simulink library "ammclib_bam_S32K14x"  (R2016a)
settings: Solver=VariableStepAuto  SolverMode=SingleTasking  StartTime=0.0  StopTime=10.0  RelTol=1e-3
undefined symbols (not defined in the file or in its folder): f16A1, f16A2, f16ADCMaxError, f16B0, f16B1, f16B2, f16C1, f16CC1, f16CC1sc, f16CC1sc_D, f16CC1sc_Q, f16CC2, f16CC2sc, f16CC2sc_D, f16CC2sc_Q, f16DerivGain, f16EGain, f16FiltCoef, f16HystOff, f16HystOn, f16IGain, f16IntegGain, f16IntegGainFW, f16IntegGainQ, f16Kd, f16Kq, f16Limit, f16LowerLimit, f16LowerLimit_D, f16LowerLimit_Q, f16LowerLimitFW, f16LowerLimitQ, f16ModIndex, f16OutValOff, f16OutValOn, f16PropGain, f16PropGainFW, f16PropGainQ, f16RampDown, f16RampUp, f16UGain, f16UpperLimit, f16UpperLimit_D, f16UpperLimit_Q, f16UpperLimitFW, f16UpperLimitQ, f16WIGain, f32A1, f32A2, f32ADCMaxError, f32B0, f32B1, f32B2, f32C1, f32CC1, f32CC1sc, f32CC1sc_D, f32CC1sc_Q, f32CC2, f32CC2sc ... (+114)
(part 15 of 22)

== system ammclib_bam_S32K14x/GMCLIB/FLT ==
  GMCLIB_BetaProjection3Ph_FLT : Subsystem  TreatAsAtomicUnit=on  mask(GMCLIB_BetaProjection3Ph_FLT){}
      mask help: 3-phase Beta-projection transformation in single precision floating-point implementation. Refer to the AMMCLIB User's Guide for further details.
      mask init: same as ammclib_bam_S32K14x/GDFLIB/F16/GDFLIB_FilterFIR_F16
      settings: RTWSystemCode=Inline
      mask Help: web([fileparts(which('ammclib_bam_S32K14x.slx')) '/../doc/S32K14XMCLUG.pdf'], '-browser')
      mask Display: pos = get_param(gcb, 'Position');width = pos(3) - pos(1); height = pos(4) - pos(2);tX=width/2;tY=height - 8;color('black');text(tX,tY, 'GMCLIB_BetaProjection3Ph_FLT', 'horizontalAlignment', 'center');
  GMCLIB_BetaProjection_FLT : Subsystem  TreatAsAtomicUnit=on  mask(GMCLIB_BetaProjection_FLT){}
      mask help: Beta Projection transformation 3ph -> 2ph in single precision floating-point implementation. Refer to the AMMCLIB User's Guide for further details.
      mask init: same as ammclib_bam_S32K14x/GDFLIB/F16/GDFLIB_FilterFIR_F16
      settings: RTWSystemCode=Inline
      mask Help: web([fileparts(which('ammclib_bam_S32K14x.slx')) '/../doc/S32K14XMCLUG.pdf'], '-browser')
      mask Display: pos = get_param(gcb, 'Position');width = pos(3) - pos(1); height = pos(4) - pos(2);tX=width/2;tY=height - 8;color('black');text(tX,tY, 'GMCLIB_BetaProjection_FLT', 'horizontalAlignment', 'center');
  GMCLIB_ClarkInv_FLT : Subsystem  TreatAsAtomicUnit=on  mask(GMCLIB_ClarkInv_FLT){}
      mask help: Inverse Clarke transformation 2ph -> 3ph in single precision floating-point implementation. Refer to the AMMCLIB User's Guide for further details.
      mask init: same as ammclib_bam_S32K14x/GDFLIB/F16/GDFLIB_FilterFIR_F16
      settings: RTWSystemCode=Inline
      mask Help: web([fileparts(which('ammclib_bam_S32K14x.slx')) '/../doc/S32K14XMCLUG.pdf'], '-browser')
      mask Display: pos = get_param(gcb, 'Position');width = pos(3) - pos(1); height = pos(4) - pos(2);tX=width/2;tY=height - 8;color('black');text(tX,tY, 'GMCLIB_ClarkInv_FLT', 'horizontalAlignment', 'center');
  GMCLIB_Clark_FLT : Subsystem  TreatAsAtomicUnit=on  mask(GMCLIB_Clark_FLT){}
      mask help: Clarke transformation 3ph -> 2ph in single precision floating-point implementation. Refer to the AMMCLIB User's Guide for further details.
      mask init: same as ammclib_bam_S32K14x/GDFLIB/F16/GDFLIB_FilterFIR_F16
      settings: RTWSystemCode=Inline
      mask Help: web([fileparts(which('ammclib_bam_S32K14x.slx')) '/../doc/S32K14XMCLUG.pdf'], '-browser')
      mask Display: pos = get_param(gcb, 'Position');width = pos(3) - pos(1); height = pos(4) - pos(2);tX=width/2;tY=height - 8;color('black');text(tX,tY, 'GMCLIB_Clark_FLT', 'horizontalAlignment', 'center');
  GMCLIB_DecouplingPMSM_FLT : Subsystem  TreatAsAtomicUnit=on  mask(GMCLIB_DecouplingPMSM_FLT){showStates=Hide (faster execution), fltLD=0, fltLQ=0}
      mask prompts: showStates "Show internal states"; fltLD "fltLD (D component of motor inductance [H])"; fltLQ "fltLQ (Q component of motor inductance [H])"
      mask help: Decoupling of d and q axis of PMSM model in single precision floating-point implementation. Refer to the AMMCLIB User's Guide for further details.
      mask init:
      | if ~evalin('base','exist(''tS8'',''var'')')
      |   if (2 ~= exist('SWLIBS_Typedefs.mat','file'))
      |       error('File SWLIBS_Typedefs.mat is not on the Matlab path. Please add the AMMCLIB "bam" folder in the Matlab Search Path.');
      |   else
      |       evalin('base', 'load(''SWLIBS_Typedefs.mat'')');
      |   end
      | end
      | if showStates == 1
      |     % hidden state variables
      |     if strcmp(get_param([gcb '/fltLD'], 'BlockType'), 'Inport')
      |         posblk = get_param(gcb, 'Position');
      | 
      |         pos = get_param(    [gcb, '/fltLD'], 'Position');
      |         orient = get_param( [gcb, '/fltLD'], 'Orientation');
      |         delete_block(       [gcb, '/fltLD']);
      |         add_block('built-in/Ground', [gcb, '/fltLD'], 'Position', pos, 'Orientation', orient);
      | 
      |         pos = get_param(    [gcb, '/fltLQ'], 'Position');
      |         orient = get_param( [gcb, '/fltLQ'], 'Orientation');
      |         delete_block(       [gcb, '/fltLQ']);
      |         add_block('built-in/Ground', [gcb, '/fltLQ'], 'Position', pos, 'Orientation', orient);
      | 
      | 
      | 
      |         set_param([gcb '/pUdq'], 'Port', '1');
      |         set_param([gcb '/pIdq'], 'Port', '2');
      |         set_param([gcb '/fltAngularVel'], 'Port', '3');
      | 
      |         set_param([gcb '/pUdqDec'], 'Port', '1');
      | 
      |         set_param(gcb,'MaskEnables',{'on','on','on'});
      | 
      |         if (posblk(4) - posblk(2)) > 100
      |           height = 100;
      |           set_param(gcb,'Position',[posblk(1), posblk(2), posblk(3), posblk(2)+height])
      |         end
      |     end
      | else
      |     % shown state variables
      |     if strcmp(get_param([gcb '/fltLD'], 'BlockType'), 'Ground')
      |         posblk = get_param(gcb, 'Position');
      | 
      |         pos = get_param(    [gcb, '/fltLD'], 'Position');
      |         orient = get_param( [gcb, '/fltLD'], 'Orientation');
      |         delete_block(       [gcb, '/fltLD']);
      |         add_block('built-in/Inport', [gcb, '/fltLD'], 'Position', pos, 'Orientation', orient, 'OutDataTypeStr', 'single');
      | 
      |         pos = get_param(    [gcb, '/fltLQ'], 'Position');
      |         orient = get_param( [gcb, '/fltLQ'], 'Orientation');
      |         delete_block(       [gcb, '/fltLQ']);
      |         add_block('built-in/Inport', [gcb, '/fltLQ'], 'Position', pos, 'Orientation', orient, 'OutDataTypeStr', 'single');
      | 
      | 
      | 
      |         set_param([gcb '/pUdq'], 'Port', '1');
      |         set_param([gcb '/pIdq'], 'Port', '2');
      |         set_param([gcb '/fltAngularVel'], 'Port', '3');
      |         set_param([gcb '/fltLD'], 'Port', '4');
      |         set_param([gcb '/fltLQ'], 'Port', '5');
      | 
      |         set_param([gcb '/pUdqDec'], 'Port', '1');
      | 
      |         set_param(gcb,'MaskEnables',{'on','off','off'});
      | 
      |         if (posblk(4) - posblk(2)) < 150
      |           height = 150;
      |           set_param(gcb,'Position',[posblk(1), posblk(2), posblk(3), posblk(2)+height])
      |         end
      |     end
      | end
      settings: RTWSystemCode=Inline
      mask Help: web([fileparts(which('ammclib_bam_S32K14x.slx')) '/../doc/S32K14XMCLUG.pdf'], '-browser')
      mask TypeOptions showStates: Hide (faster execution) | Show (allows debugging; connect feedback loops manually)
      mask Callback showStates:
      | maskStr = get_param(gcb,'showStates');
      | if strcmp(maskStr,'Hide (faster execution)'),
      |     set_param(gcb,'MaskEnables',{'on','on','on'});
      | else
      |     set_param(gcb,'MaskEnables',{'on','off','off'});
      | end
      mask Display:
      | color('black');
      | pos = get_param(gcb, 'Position');
      | width = pos(3) - pos(1);
      | height = pos(4) - pos(2);
      | tX=width/2;
      | tY=height - 8;
      | color('black');
      | text(tX,tY, 'GMCLIB_DecouplingPMSM_FLT', 'horizontalAlignment', 'center');
      | if showStates == 2
      |   color('red');
      |   text(tX,tY - 20, ['debugging mode' char(13) char(10) '(limited performance)'], 'horizontalAlignment', 'center');
      | end
  GMCLIB_ElimDcBusRip_FLT : Subsystem  TreatAsAtomicUnit=on  mask(GMCLIB_ElimDcBusRip_FLT){showStates=Hide (faster execution), fltModIndex=0}
      mask prompts: showStates "Show internal states"; fltModIndex "fltModIndex (Inverse Modulation Index)"
      mask help: DC Bus voltage ripple elimination function in single precision floating-point implementation. Refer to the AMMCLIB User's Guide for further details.
      mask init:
      | if ~evalin('base','exist(''tS8'',''var'')')
      |   if (2 ~= exist('SWLIBS_Typedefs.mat','file'))
      |       error('File SWLIBS_Typedefs.mat is not on the Matlab path. Please add the AMMCLIB "bam" folder in the Matlab Search Path.');
      |   else
      |       evalin('base', 'load(''SWLIBS_Typedefs.mat'')');
      |   end
      | end
      | if showStates == 1
      |     % hidden state variables
      |     if strcmp(get_param([gcb '/fltModIndex'], 'BlockType'), 'Inport')
      |         posblk = get_param(gcb, 'Position');
      | 
      |         pos = get_param(    [gcb, '/fltModIndex'], 'Position');
      |         orient = get_param( [gcb, '/fltModIndex'], 'Orientation');
      |         delete_block(       [gcb, '/fltModIndex']);
      |         add_block('built-in/Ground', [gcb, '/fltModIndex'], 'Position', pos, 'Orientation', orient);
      | 
      | 
      | 
      |         set_param([gcb '/pIn'], 'Port', '1');
      |         set_param([gcb '/fltArgDcBusMsr'], 'Port', '2');
      | 
      |         set_param([gcb '/pOut'], 'Port', '1');
      | 
      |         set_param(gcb,'MaskEnables',{'on','on'});
      | 
      |         if (posblk(4) - posblk(2)) > 75
      |           height = 75;
      |           set_param(gcb,'Position',[posblk(1), posblk(2), posblk(3), posblk(2)+height])
      |         end
      |     end
      | else
      |     % shown state variables
      |     if strcmp(get_param([gcb '/fltModIndex'], 'BlockType'), 'Ground')
      |         posblk = get_param(gcb, 'Position');
      | 
      |         pos = get_param(    [gcb, '/fltModIndex'], 'Position');
      |         orient = get_param( [gcb, '/fltModIndex'], 'Orientation');
      |         delete_block(       [gcb, '/fltModIndex']);
      |         add_block('built-in/Inport', [gcb, '/fltModIndex'], 'Position', pos, 'Orientation', orient, 'OutDataTypeStr', 'single');
      | 
      | 
      | 
      |         set_param([gcb '/pIn'], 'Port', '1');
      |         set_param([gcb '/fltArgDcBusMsr'], 'Port', '2');
      |         set_param([gcb '/fltModIndex'], 'Port', '3');
      | 
      |         set_param([gcb '/pOut'], 'Port', '1');
      | 
      |         set_param(gcb,'MaskEnables',{'on','off'});
      | 
      |         if (posblk(4) - posblk(2)) < 100
      |           height = 100;
      |           set_param(gcb,'Position',[posblk(1), posblk(2), posblk(3), posblk(2)+height])
      |         end
      |     end
      | end
      settings: RTWSystemCode=Inline
      mask Help: web([fileparts(which('ammclib_bam_S32K14x.slx')) '/../doc/S32K14XMCLUG.pdf'], '-browser')
      mask TypeOptions showStates: Hide (faster execution) | Show (allows debugging; connect feedback loops manually)
      mask Callback showStates:
      | maskStr = get_param(gcb,'showStates');
      | if strcmp(maskStr,'Hide (faster execution)'),
      |     set_param(gcb,'MaskEnables',{'on','on'});
      | else
      |     set_param(gcb,'MaskEnables',{'on','off'});
      | end
      mask Display:
      | color('black');
      | pos = get_param(gcb, 'Position');
      | width = pos(3) - pos(1);
      | height = pos(4) - pos(2);
      | tX=width/2;
      | tY=height - 8;
      | color('black');
      | text(tX,tY, 'GMCLIB_ElimDcBusRip_FLT', 'horizontalAlignment', 'center');
      | if showStates == 2
      |   color('red');
      |   text(tX,tY - 20, ['debugging mode' char(13) char(10) '(limited performance)'], 'horizontalAlignment', 'center');
      | end
  GMCLIB_ParkInv_FLT : Subsystem  TreatAsAtomicUnit=on  mask(GMCLIB_ParkInv_FLT){}
      mask help: Inverse Park transformation 2ph rotational -> 2ph stationary in single precision floating-point implementation. Refer to the AMMCLIB User's Guide for further details.
      mask init: same as ammclib_bam_S32K14x/GDFLIB/F16/GDFLIB_FilterFIR_F16
      settings: RTWSystemCode=Inline
      mask Help: web([fileparts(which('ammclib_bam_S32K14x.slx')) '/../doc/S32K14XMCLUG.pdf'], '-browser')
      mask Display: pos = get_param(gcb, 'Position');width = pos(3) - pos(1); height = pos(4) - pos(2);tX=width/2;tY=height - 8;color('black');text(tX,tY, 'GMCLIB_ParkInv_FLT', 'horizontalAlignment', 'center');
  GMCLIB_Park_FLT : Subsystem  TreatAsAtomicUnit=on  mask(GMCLIB_Park_FLT){}
      mask help: Park transformation 2ph stationary -> 2ph rotational in single precision floating-point implementation. Refer to the AMMCLIB User's Guide for further details.
      mask init: same as ammclib_bam_S32K14x/GDFLIB/F16/GDFLIB_FilterFIR_F16
      settings: RTWSystemCode=Inline
      mask Help: web([fileparts(which('ammclib_bam_S32K14x.slx')) '/../doc/S32K14XMCLUG.pdf'], '-browser')
      mask Display: pos = get_param(gcb, 'Position');width = pos(3) - pos(1); height = pos(4) - pos(2);tX=width/2;tY=height - 8;color('black');text(tX,tY, 'GMCLIB_Park_FLT', 'horizontalAlignment', 'center');
  GMCLIB_PwmIct_FLT : Subsystem  TreatAsAtomicUnit=on  mask(GMCLIB_PwmIct_FLT){}
      mask help: General Sinusoidal PWM in single precision floating-point implementation. Refer to the AMMCLIB User's Guide for further details.
      mask init: same as ammclib_bam_S32K14x/GDFLIB/F16/GDFLIB_FilterFIR_F16
      settings: RTWSystemCode=Inline
      mask Help: web([fileparts(which('ammclib_bam_S32K14x.slx')) '/../doc/S32K14XMCLUG.pdf'], '-browser')
      mask Display: pos = get_param(gcb, 'Position');width = pos(3) - pos(1); height = pos(4) - pos(2);tX=width/2;tY=height - 8;color('black');text(tX,tY, 'GMCLIB_PwmIct_FLT', 'horizontalAlignment', 'center');
  GMCLIB_SvmSci_FLT : Subsystem  TreatAsAtomicUnit=on  mask(GMCLIB_SvmSci_FLT){}
      mask help: General Sinusoidal Modulation with Injection of Third Harmonic in single precision floating-point implementation. Refer to the AMMCLIB User's Guide for further details.
      mask init: same as ammclib_bam_S32K14x/GDFLIB/F16/GDFLIB_FilterFIR_F16
      settings: RTWSystemCode=Inline
      mask Help: web([fileparts(which('ammclib_bam_S32K14x.slx')) '/../doc/S32K14XMCLUG.pdf'], '-browser')
      mask Display: pos = get_param(gcb, 'Position');width = pos(3) - pos(1); height = pos(4) - pos(2);tX=width/2;tY=height - 8;color('black');text(tX,tY, 'GMCLIB_SvmSci_FLT', 'horizontalAlignment', 'center');
  GMCLIB_SvmStd_FLT : Subsystem  TreatAsAtomicUnit=on  mask(GMCLIB_SvmStd_FLT){}
      mask help: Standard Space Vector Modulation in single precision floating-point implementation. Refer to the AMMCLIB User's Guide for further details.
      mask init: same as ammclib_bam_S32K14x/GDFLIB/F16/GDFLIB_FilterFIR_F16
      settings: RTWSystemCode=Inline
      mask Help: web([fileparts(which('ammclib_bam_S32K14x.slx')) '/../doc/S32K14XMCLUG.pdf'], '-browser')
      mask Display: pos = get_param(gcb, 'Position');width = pos(3) - pos(1); height = pos(4) - pos(2);tX=width/2;tY=height - 8;color('black');text(tX,tY, 'GMCLIB_SvmStd_FLT', 'horizontalAlignment', 'center');
  GMCLIB_SvmU0n_FLT : Subsystem  TreatAsAtomicUnit=on  mask(GMCLIB_SvmU0n_FLT){}
      mask help: Special Space Vector Modulation with O_000 Nulls in single precision floating-point implementation. Refer to the AMMCLIB User's Guide for further details.
      mask init: same as ammclib_bam_S32K14x/GDFLIB/F16/GDFLIB_FilterFIR_F16
      settings: RTWSystemCode=Inline
      mask Help: web([fileparts(which('ammclib_bam_S32K14x.slx')) '/../doc/S32K14XMCLUG.pdf'], '-browser')
      mask Display: pos = get_param(gcb, 'Position');width = pos(3) - pos(1); height = pos(4) - pos(2);tX=width/2;tY=height - 8;color('black');text(tX,tY, 'GMCLIB_SvmU0n_FLT', 'horizontalAlignment', 'center');
  GMCLIB_SvmU7n_FLT : Subsystem  TreatAsAtomicUnit=on  mask(GMCLIB_SvmU7n_FLT){}
      mask help: Special Space Vector Modulation with O_111 Ones in single precision floating-point implementation. Refer to the AMMCLIB User's Guide for further details.
      mask init: same as ammclib_bam_S32K14x/GDFLIB/F16/GDFLIB_FilterFIR_F16
      settings: RTWSystemCode=Inline
      mask Help: web([fileparts(which('ammclib_bam_S32K14x.slx')) '/../doc/S32K14XMCLUG.pdf'], '-browser')
      mask Display: pos = get_param(gcb, 'Position');width = pos(3) - pos(1); height = pos(4) - pos(2);tX=width/2;tY=height - 8;color('black');text(tX,tY, 'GMCLIB_SvmU7n_FLT', 'horizontalAlignment', 'center');
  GMCLIB_VRot_FLT : Subsystem  TreatAsAtomicUnit=on  mask(GMCLIB_VRot_FLT){}
      mask help: Vector rotation in single precision floating-point implementation.
      mask init: same as ammclib_bam_S32K14x/GDFLIB/F16/GDFLIB_FilterFIR_F16
      settings: RTWSystemCode=Inline
      mask Help: web([fileparts(which('ammclib_bam_S32K14x.slx')) '/../doc/S32K14XMCLUG.pdf'], '-browser')
      mask Display: pos = get_param(gcb, 'Position');width = pos(3) - pos(1); height = pos(4) - pos(2);tX=width/2;tY=height - 8;color('black');text(tX,tY, 'GMCLIB_VRot_FLT', 'horizontalAlignment', 'center');
  GMCLIB_VUnit_FLT : Subsystem  TreatAsAtomicUnit=on  mask(GMCLIB_VUnit_FLT){}
      mask help: Vector normalization in single precision floating-point implementation.
      mask init: same as ammclib_bam_S32K14x/GDFLIB/F16/GDFLIB_FilterFIR_F16
      settings: RTWSystemCode=Inline
      mask Help: web([fileparts(which('ammclib_bam_S32K14x.slx')) '/../doc/S32K14XMCLUG.pdf'], '-browser')
      mask Display: pos = get_param(gcb, 'Position');width = pos(3) - pos(1); height = pos(4) - pos(2);tX=width/2;tY=height - 8;color('black');text(tX,tY, 'GMCLIB_VUnit_FLT', 'horizontalAlignment', 'center');
  GMCLIB_Vpol2xy_FLT : Subsystem  TreatAsAtomicUnit=on  mask(GMCLIB_Vpol2xy_FLT){}
      mask help: Transformation of polar coordinate system to Cartesian in single precision floating-point implementation.
      mask init: same as ammclib_bam_S32K14x/GDFLIB/F16/GDFLIB_FilterFIR_F16
      settings: RTWSystemCode=Inline
      mask Help: web([fileparts(which('ammclib_bam_S32K14x.slx')) '/../doc/S32K14XMCLUG.pdf'], '-browser')
      mask Display: pos = get_param(gcb, 'Position');width = pos(3) - pos(1); height = pos(4) - pos(2);tX=width/2;tY=height - 8;color('black');text(tX,tY, 'GMCLIB_Vpol2xy_FLT', 'horizontalAlignment', 'center');
  GMCLIB_Vxy2pol_FLT : Subsystem  TreatAsAtomicUnit=on  mask(GMCLIB_Vxy2pol_FLT){}
      mask help: Transformation of Cartesian coordinate system to polar in single precision floating-point implementation.
      mask init: same as ammclib_bam_S32K14x/GDFLIB/F16/GDFLIB_FilterFIR_F16
      settings: RTWSystemCode=Inline
      mask Help: web([fileparts(which('ammclib_bam_S32K14x.slx')) '/../doc/S32K14XMCLUG.pdf'], '-browser')
      mask Display: pos = get_param(gcb, 'Position');width = pos(3) - pos(1); height = pos(4) - pos(2);tX=width/2;tY=height - 8;color('black');text(tX,tY, 'GMCLIB_Vxy2pol_FLT', 'horizontalAlignment', 'center');

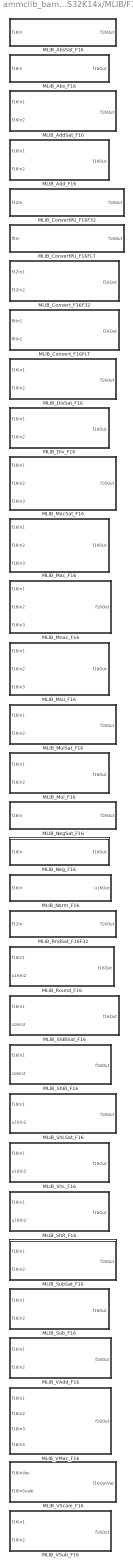
== system ammclib_bam_S32K14x/MLIB/F16 ==
  MLIB_AbsSat_F16 : Subsystem  TreatAsAtomicUnit=on  mask(MLIB_AbsSat_F16){}
      mask help: Saturated absolute value in 16-bit fixed-point fractional implementation. Refer to the AMMCLIB User's Guide for further details.
      mask init: same as ammclib_bam_S32K14x/GDFLIB/F16/GDFLIB_FilterFIR_F16
      settings: RTWSystemCode=Inline
      mask Help: web([fileparts(which('ammclib_bam_S32K14x.slx')) '/../doc/S32K14XMCLUG.pdf'], '-browser')
      mask Display: pos = get_param(gcb, 'Position');width = pos(3) - pos(1); height = pos(4) - pos(2);tX=width/2;tY=height - 8;color('black');text(tX,tY, 'MLIB_AbsSat_F16', 'horizontalAlignment', 'center');
  MLIB_Abs_F16 : Subsystem  TreatAsAtomicUnit=on  mask(MLIB_Abs_F16){}
      mask help: Unsaturated absolute value in 16-bit fixed-point fractional implementation. Refer to the AMMCLIB User's Guide for further details.
      mask init: same as ammclib_bam_S32K14x/GDFLIB/F16/GDFLIB_FilterFIR_F16
      settings: RTWSystemCode=Inline
      mask Help: web([fileparts(which('ammclib_bam_S32K14x.slx')) '/../doc/S32K14XMCLUG.pdf'], '-browser')
      mask Display: pos = get_param(gcb, 'Position');width = pos(3) - pos(1); height = pos(4) - pos(2);tX=width/2;tY=height - 8;color('black');text(tX,tY, 'MLIB_Abs_F16', 'horizontalAlignment', 'center');
  MLIB_AddSat_F16 : Subsystem  TreatAsAtomicUnit=on  mask(MLIB_AddSat_F16){}
      mask help: Saturated addition in 16-bit fixed-point fractional implementation. Refer to the AMMCLIB User's Guide for further details.
      mask init: same as ammclib_bam_S32K14x/GDFLIB/F16/GDFLIB_FilterFIR_F16
      settings: RTWSystemCode=Inline
      mask Help: web([fileparts(which('ammclib_bam_S32K14x.slx')) '/../doc/S32K14XMCLUG.pdf'], '-browser')
      mask Display: pos = get_param(gcb, 'Position');width = pos(3) - pos(1); height = pos(4) - pos(2);tX=width/2;tY=height - 8;color('black');text(tX,tY, 'MLIB_AddSat_F16', 'horizontalAlignment', 'center');
  MLIB_Add_F16 : Subsystem  TreatAsAtomicUnit=on  mask(MLIB_Add_F16){}
      mask help: Unsaturated addition in 16-bit fixed-point fractional implementation.
      mask init: same as ammclib_bam_S32K14x/GDFLIB/F16/GDFLIB_FilterFIR_F16
      settings: RTWSystemCode=Inline
      mask Help: web([fileparts(which('ammclib_bam_S32K14x.slx')) '/../doc/S32K14XMCLUG.pdf'], '-browser')
      mask Display: pos = get_param(gcb, 'Position');width = pos(3) - pos(1); height = pos(4) - pos(2);tX=width/2;tY=height - 8;color('black');text(tX,tY, 'MLIB_Add_F16', 'horizontalAlignment', 'center');
  MLIB_ConvertPU_F16F32 : Subsystem  TreatAsAtomicUnit=on  mask(MLIB_ConvertPU_F16F32){}
      mask help: Conversion of a 32-bit fixed-point fractional value to a 16-bit fixed-point fractional equivalent. Refer to the AMMCLIB User's Guide for further details.
      mask init: same as ammclib_bam_S32K14x/GDFLIB/F16/GDFLIB_FilterFIR_F16
      settings: RTWSystemCode=Inline
      mask Help: web([fileparts(which('ammclib_bam_S32K14x.slx')) '/../doc/S32K14XMCLUG.pdf'], '-browser')
      mask Display: pos = get_param(gcb, 'Position');width = pos(3) - pos(1); height = pos(4) - pos(2);tX=width/2;tY=height - 8;color('black');text(tX,tY, 'MLIB_ConvertPU_F16F32', 'horizontalAlignment', 'center');
  MLIB_ConvertPU_F16FLT : Subsystem  TreatAsAtomicUnit=on  mask(MLIB_ConvertPU_F16FLT){}
      mask help: Conversion of a single precision floating-point value to a 16-bit fixed-point fractional equivalent. Refer to the AMMCLIB User's Guide for further details.
      mask init: same as ammclib_bam_S32K14x/GDFLIB/F16/GDFLIB_FilterFIR_F16
      settings: RTWSystemCode=Inline
      mask Help: web([fileparts(which('ammclib_bam_S32K14x.slx')) '/../doc/S32K14XMCLUG.pdf'], '-browser')
      mask Display: pos = get_param(gcb, 'Position');width = pos(3) - pos(1); height = pos(4) - pos(2);tX=width/2;tY=height - 8;color('black');text(tX,tY, 'MLIB_ConvertPU_F16FLT', 'horizontalAlignment', 'center');
  MLIB_Convert_F16F32 : Subsystem  TreatAsAtomicUnit=on  mask(MLIB_Convert_F16F32){}
      mask help: Scaled conversion of a 32-bit fixed-point fractional value to a 16-bit fixed-point fractional equivalent. Refer to the AMMCLIB User's Guide for further details.
      mask init: same as ammclib_bam_S32K14x/GDFLIB/F16/GDFLIB_FilterFIR_F16
      settings: RTWSystemCode=Inline
      mask Help: web([fileparts(which('ammclib_bam_S32K14x.slx')) '/../doc/S32K14XMCLUG.pdf'], '-browser')
      mask Display: pos = get_param(gcb, 'Position');width = pos(3) - pos(1); height = pos(4) - pos(2);tX=width/2;tY=height - 8;color('black');text(tX,tY, 'MLIB_Convert_F16F32', 'horizontalAlignment', 'center');
  MLIB_Convert_F16FLT : Subsystem  TreatAsAtomicUnit=on  mask(MLIB_Convert_F16FLT){}
      mask help: Scaled conversion of a single precision floating-point value to a 16-bit fixed-point fractional equivalent. Refer to the AMMCLIB User's Guide for further details.
      mask init: same as ammclib_bam_S32K14x/GDFLIB/F16/GDFLIB_FilterFIR_F16
      settings: RTWSystemCode=Inline
      mask Help: web([fileparts(which('ammclib_bam_S32K14x.slx')) '/../doc/S32K14XMCLUG.pdf'], '-browser')
      mask Display: pos = get_param(gcb, 'Position');width = pos(3) - pos(1); height = pos(4) - pos(2);tX=width/2;tY=height - 8;color('black');text(tX,tY, 'MLIB_Convert_F16FLT', 'horizontalAlignment', 'center');
  MLIB_DivSat_F16 : Subsystem  TreatAsAtomicUnit=on  mask(MLIB_DivSat_F16){}
      mask help: Saturated division of two input values in 16-bit fixed-point fractional implementation. Refer to the AMMCLIB User's Guide for further details.
      mask init: same as ammclib_bam_S32K14x/GDFLIB/F16/GDFLIB_FilterFIR_F16
      settings: RTWSystemCode=Inline
      mask Help: web([fileparts(which('ammclib_bam_S32K14x.slx')) '/../doc/S32K14XMCLUG.pdf'], '-browser')
      mask Display: pos = get_param(gcb, 'Position');width = pos(3) - pos(1); height = pos(4) - pos(2);tX=width/2;tY=height - 8;color('black');text(tX,tY, 'MLIB_DivSat_F16', 'horizontalAlignment', 'center');
  MLIB_Div_F16 : Subsystem  TreatAsAtomicUnit=on  mask(MLIB_Div_F16){}
      mask help: Division of two input values without saturation in 16-bit fixed-point fractional implementation. Refer to the AMMCLIB User's Guide for further details.
      mask init: same as ammclib_bam_S32K14x/GDFLIB/F16/GDFLIB_FilterFIR_F16
      settings: RTWSystemCode=Inline
      mask Help: web([fileparts(which('ammclib_bam_S32K14x.slx')) '/../doc/S32K14XMCLUG.pdf'], '-browser')
      mask Display: pos = get_param(gcb, 'Position');width = pos(3) - pos(1); height = pos(4) - pos(2);tX=width/2;tY=height - 8;color('black');text(tX,tY, 'MLIB_Div_F16', 'horizontalAlignment', 'center');
  MLIB_MacSat_F16 : Subsystem  TreatAsAtomicUnit=on  mask(MLIB_MacSat_F16){}
      mask help: Saturated multiply-accumulate of input values in 16-bit fixed-point fractional implementation. Refer to the AMMCLIB User's Guide for further details.
      mask init: same as ammclib_bam_S32K14x/GDFLIB/F16/GDFLIB_FilterFIR_F16
      settings: RTWSystemCode=Inline
      mask Help: web([fileparts(which('ammclib_bam_S32K14x.slx')) '/../doc/S32K14XMCLUG.pdf'], '-browser')
      mask Display: pos = get_param(gcb, 'Position');width = pos(3) - pos(1); height = pos(4) - pos(2);tX=width/2;tY=height - 8;color('black');text(tX,tY, 'MLIB_MacSat_F16', 'horizontalAlignment', 'center');
  MLIB_Mac_F16 : Subsystem  TreatAsAtomicUnit=on  mask(MLIB_Mac_F16){}
      mask help: Unsaturated multiply-accumulate function in 16-bit fixed-point fractional implementation. Refer to the AMMCLIB User's Guide for further details.
      mask init: same as ammclib_bam_S32K14x/GDFLIB/F16/GDFLIB_FilterFIR_F16
      settings: RTWSystemCode=Inline
      mask Help: web([fileparts(which('ammclib_bam_S32K14x.slx')) '/../doc/S32K14XMCLUG.pdf'], '-browser')
      mask Display: pos = get_param(gcb, 'Position');width = pos(3) - pos(1); height = pos(4) - pos(2);tX=width/2;tY=height - 8;color('black');text(tX,tY, 'MLIB_Mac_F16', 'horizontalAlignment', 'center');
  MLIB_Mnac_F16 : Subsystem  TreatAsAtomicUnit=on  mask(MLIB_Mnac_F16){}
      mask help: Unsaturated multiply-negative-accumulate function in 16-bit fixed-point fractional implementation. Refer to the AMMCLIB User's Guide for further details.
      mask init: same as ammclib_bam_S32K14x/GDFLIB/F16/GDFLIB_FilterFIR_F16
      settings: RTWSystemCode=Inline
      mask Help: web([fileparts(which('ammclib_bam_S32K14x.slx')) '/../doc/S32K14XMCLUG.pdf'], '-browser')
      mask Display: pos = get_param(gcb, 'Position');width = pos(3) - pos(1); height = pos(4) - pos(2);tX=width/2;tY=height - 8;color('black');text(tX,tY, 'MLIB_Mnac_F16', 'horizontalAlignment', 'center');
  MLIB_Msu_F16 : Subsystem  TreatAsAtomicUnit=on  mask(MLIB_Msu_F16){}
      mask help: Unsaturated multiply-subtract-from function in 16-bit fixed-point fractional implementation. Refer to the AMMCLIB User's Guide for further details.
      mask init: same as ammclib_bam_S32K14x/GDFLIB/F16/GDFLIB_FilterFIR_F16
      settings: RTWSystemCode=Inline
      mask Help: web([fileparts(which('ammclib_bam_S32K14x.slx')) '/../doc/S32K14XMCLUG.pdf'], '-browser')
      mask Display: pos = get_param(gcb, 'Position');width = pos(3) - pos(1); height = pos(4) - pos(2);tX=width/2;tY=height - 8;color('black');text(tX,tY, 'MLIB_Msu_F16', 'horizontalAlignment', 'center');
  MLIB_MulSat_F16 : Subsystem  TreatAsAtomicUnit=on  mask(MLIB_MulSat_F16){}
      mask help: Saturated multiplication of two input values in 16-bit fixed-point fractional implementation. Refer to the AMMCLIB User's Guide for further details.
      mask init: same as ammclib_bam_S32K14x/GDFLIB/F16/GDFLIB_FilterFIR_F16
      settings: RTWSystemCode=Inline
      mask Help: web([fileparts(which('ammclib_bam_S32K14x.slx')) '/../doc/S32K14XMCLUG.pdf'], '-browser')
      mask Display: pos = get_param(gcb, 'Position');width = pos(3) - pos(1); height = pos(4) - pos(2);tX=width/2;tY=height - 8;color('black');text(tX,tY, 'MLIB_MulSat_F16', 'horizontalAlignment', 'center');
  MLIB_Mul_F16 : Subsystem  TreatAsAtomicUnit=on  mask(MLIB_Mul_F16){}
      mask help: Unsaturated multiplication of two input values in 16-bit fixed-point fractional implementation. Refer to the AMMCLIB User's Guide for further details.
      mask init: same as ammclib_bam_S32K14x/GDFLIB/F16/GDFLIB_FilterFIR_F16
      settings: RTWSystemCode=Inline
      mask Help: web([fileparts(which('ammclib_bam_S32K14x.slx')) '/../doc/S32K14XMCLUG.pdf'], '-browser')
      mask Display: pos = get_param(gcb, 'Position');width = pos(3) - pos(1); height = pos(4) - pos(2);tX=width/2;tY=height - 8;color('black');text(tX,tY, 'MLIB_Mul_F16', 'horizontalAlignment', 'center');
  MLIB_NegSat_F16 : Subsystem  TreatAsAtomicUnit=on  mask(MLIB_NegSat_F16){}
      mask help: Saturated negation in 16-bit fixed-point fractional implementation. Refer to the AMMCLIB User's Guide for further details.
      mask init: same as ammclib_bam_S32K14x/GDFLIB/F16/GDFLIB_FilterFIR_F16
      settings: RTWSystemCode=Inline
      mask Help: web([fileparts(which('ammclib_bam_S32K14x.slx')) '/../doc/S32K14XMCLUG.pdf'], '-browser')
      mask Display: pos = get_param(gcb, 'Position');width = pos(3) - pos(1); height = pos(4) - pos(2);tX=width/2;tY=height - 8;color('black');text(tX,tY, 'MLIB_NegSat_F16', 'horizontalAlignment', 'center');
  MLIB_Neg_F16 : Subsystem  TreatAsAtomicUnit=on  mask(MLIB_Neg_F16){}
      mask help: Unsaturated negation in 16-bit fixed-point fractional implementation. Refer to the AMMCLIB User's Guide for further details.
      mask init: same as ammclib_bam_S32K14x/GDFLIB/F16/GDFLIB_FilterFIR_F16
      settings: RTWSystemCode=Inline
      mask Help: web([fileparts(which('ammclib_bam_S32K14x.slx')) '/../doc/S32K14XMCLUG.pdf'], '-browser')
      mask Display: pos = get_param(gcb, 'Position');width = pos(3) - pos(1); height = pos(4) - pos(2);tX=width/2;tY=height - 8;color('black');text(tX,tY, 'MLIB_Neg_F16', 'horizontalAlignment', 'center');
  MLIB_Norm_F16 : Subsystem  TreatAsAtomicUnit=on  mask(MLIB_Norm_F16){}
      mask help: Normalization function in 16-bit fixed-point fractional implementation. The function counts the number of left shift needed for normalization of the input fractional value. Refer to the AMMCLIB User's Guide for further details.
      mask init: same as ammclib_bam_S32K14x/GDFLIB/F16/GDFLIB_FilterFIR_F16
      settings: RTWSystemCode=Inline
      mask Help: web([fileparts(which('ammclib_bam_S32K14x.slx')) '/../doc/S32K14XMCLUG.pdf'], '-browser')
      mask Display: pos = get_param(gcb, 'Position');width = pos(3) - pos(1); height = pos(4) - pos(2);tX=width/2;tY=height - 8;color('black');text(tX,tY, 'MLIB_Norm_F16', 'horizontalAlignment', 'center');
  MLIB_RndSat_F16F32 : Subsystem  TreatAsAtomicUnit=on  mask(MLIB_RndSat_F16F32){}
      mask help: Saturated round to the nearest 16-bit fractional value. Refer to the AMMCLIB User's Guide for further details.
      mask init: same as ammclib_bam_S32K14x/GDFLIB/F16/GDFLIB_FilterFIR_F16
      settings: RTWSystemCode=Inline
      mask Help: web([fileparts(which('ammclib_bam_S32K14x.slx')) '/../doc/S32K14XMCLUG.pdf'], '-browser')
      mask Display: pos = get_param(gcb, 'Position');width = pos(3) - pos(1); height = pos(4) - pos(2);tX=width/2;tY=height - 8;color('black');text(tX,tY, 'MLIB_RndSat_F16F32', 'horizontalAlignment', 'center');
  MLIB_Round_F16 : Subsystem  TreatAsAtomicUnit=on  mask(MLIB_Round_F16){}
      mask help: Rounding function in 16-bit fixed-point fractional implementation. The function rounds the first input value to the number of digits defined by second input value and saturates the result. Refer to the AMMCLIB User's Guide for further details.
      mask init: same as ammclib_bam_S32K14x/GDFLIB/F16/GDFLIB_FilterFIR_F16
      settings: RTWSystemCode=Inline
      mask Help: web([fileparts(which('ammclib_bam_S32K14x.slx')) '/../doc/S32K14XMCLUG.pdf'], '-browser')
      mask Display: pos = get_param(gcb, 'Position');width = pos(3) - pos(1); height = pos(4) - pos(2);tX=width/2;tY=height - 8;color('black');text(tX,tY, 'MLIB_Round_F16', 'horizontalAlignment', 'center');
  MLIB_ShBiSat_F16 : Subsystem  TreatAsAtomicUnit=on  mask(MLIB_ShBiSat_F16){}
      mask help: Saturated bidirectional shift in 16-bit fixed-point fractional implementation. The function shifts the first input value to the left (if the second input is negative) or right (if the second input is positive) by the amount defined by second input value, saturating the result. Refer to the AMMCLIB User's Guide for further details.
      mask init: same as ammclib_bam_S32K14x/GDFLIB/F16/GDFLIB_FilterFIR_F16
      settings: RTWSystemCode=Inline
      mask Help: web([fileparts(which('ammclib_bam_S32K14x.slx')) '/../doc/S32K14XMCLUG.pdf'], '-browser')
      mask Display: pos = get_param(gcb, 'Position');width = pos(3) - pos(1); height = pos(4) - pos(2);tX=width/2;tY=height - 8;color('black');text(tX,tY, 'MLIB_ShBiSat_F16', 'horizontalAlignment', 'center');
  MLIB_ShBi_F16 : Subsystem  TreatAsAtomicUnit=on  mask(MLIB_ShBi_F16){}
      mask help: Unsaturated bidirectional shift in 16-bit fixed-point fractional implementation. The function shifts the first input value to the left (if the second input is negative) or right (if the second input is positive) by the amount defined by second input value. Refer to the AMMCLIB User's Guide for further details.
      mask init: same as ammclib_bam_S32K14x/GDFLIB/F16/GDFLIB_FilterFIR_F16
      settings: RTWSystemCode=Inline
      mask Help: web([fileparts(which('ammclib_bam_S32K14x.slx')) '/../doc/S32K14XMCLUG.pdf'], '-browser')
      mask Display: pos = get_param(gcb, 'Position');width = pos(3) - pos(1); height = pos(4) - pos(2);tX=width/2;tY=height - 8;color('black');text(tX,tY, 'MLIB_ShBi_F16', 'horizontalAlignment', 'center');
  MLIB_ShLSat_F16 : Subsystem  TreatAsAtomicUnit=on  mask(MLIB_ShLSat_F16){}
      mask help: Saturated shift left in 16-bit fixed-point fractional implementation. The function shifts the first input value to the left by the amount defined by the second input value, saturating the result. Refer to the AMMCLIB User's Guide for further details.
      mask init: same as ammclib_bam_S32K14x/GDFLIB/F16/GDFLIB_FilterFIR_F16
      settings: RTWSystemCode=Inline
      mask Help: web([fileparts(which('ammclib_bam_S32K14x.slx')) '/../doc/S32K14XMCLUG.pdf'], '-browser')
      mask Display: pos = get_param(gcb, 'Position');width = pos(3) - pos(1); height = pos(4) - pos(2);tX=width/2;tY=height - 8;color('black');text(tX,tY, 'MLIB_ShLSat_F16', 'horizontalAlignment', 'center');
  MLIB_ShL_F16 : Subsystem  TreatAsAtomicUnit=on  mask(MLIB_ShL_F16){}
      mask help: Unsaturated shift left in 16-bit fixed-point fractional implementation. The function shifts the first input value to the left by the amount defined by the second input value. Refer to the AMMCLIB User's Guide for further details.
      mask init: same as ammclib_bam_S32K14x/GDFLIB/F16/GDFLIB_FilterFIR_F16
      settings: RTWSystemCode=Inline
      mask Help: web([fileparts(which('ammclib_bam_S32K14x.slx')) '/../doc/S32K14XMCLUG.pdf'], '-browser')
      mask Display: pos = get_param(gcb, 'Position');width = pos(3) - pos(1); height = pos(4) - pos(2);tX=width/2;tY=height - 8;color('black');text(tX,tY, 'MLIB_ShL_F16', 'horizontalAlignment', 'center');
  MLIB_ShR_F16 : Subsystem  TreatAsAtomicUnit=on  mask(MLIB_ShR_F16){}
      mask help: Unsaturated shift right in 16-bit fixed-point fractional implementation. The function shifts the first input value to the right by the amount defined by the second input value. Refer to the AMMCLIB User's Guide for further details.
      mask init: same as ammclib_bam_S32K14x/GDFLIB/F16/GDFLIB_FilterFIR_F16
      settings: RTWSystemCode=Inline
      mask Help: web([fileparts(which('ammclib_bam_S32K14x.slx')) '/../doc/S32K14XMCLUG.pdf'], '-browser')
      mask Display: pos = get_param(gcb, 'Position');width = pos(3) - pos(1); height = pos(4) - pos(2);tX=width/2;tY=height - 8;color('black');text(tX,tY, 'MLIB_ShR_F16', 'horizontalAlignment', 'center');
  MLIB_SubSat_F16 : Subsystem  TreatAsAtomicUnit=on  mask(MLIB_SubSat_F16){}
      mask help: Saturated subtraction in 16-bit fixed-point fractional implementation. Refer to the AMMCLIB User's Guide for further details.
      mask init: same as ammclib_bam_S32K14x/GDFLIB/F16/GDFLIB_FilterFIR_F16
      settings: RTWSystemCode=Inline
      mask Help: web([fileparts(which('ammclib_bam_S32K14x.slx')) '/../doc/S32K14XMCLUG.pdf'], '-browser')
      mask Display: pos = get_param(gcb, 'Position');width = pos(3) - pos(1); height = pos(4) - pos(2);tX=width/2;tY=height - 8;color('black');text(tX,tY, 'MLIB_SubSat_F16', 'horizontalAlignment', 'center');
  MLIB_Sub_F16 : Subsystem  TreatAsAtomicUnit=on  mask(MLIB_Sub_F16){}
      mask help: Unsaturated subtraction in 16-bit fixed-point fractional implementation. Refer to the AMMCLIB User's Guide for further details.
      mask init: same as ammclib_bam_S32K14x/GDFLIB/F16/GDFLIB_FilterFIR_F16
      settings: RTWSystemCode=Inline
      mask Help: web([fileparts(which('ammclib_bam_S32K14x.slx')) '/../doc/S32K14XMCLUG.pdf'], '-browser')
      mask Display: pos = get_param(gcb, 'Position');width = pos(3) - pos(1); height = pos(4) - pos(2);tX=width/2;tY=height - 8;color('black');text(tX,tY, 'MLIB_Sub_F16', 'horizontalAlignment', 'center');
  MLIB_VAdd_F16 : Subsystem  TreatAsAtomicUnit=on  mask(MLIB_VAdd_F16){}
      mask help: Vector addition in 16-bit fixed-point fractional implementation.
      mask init: same as ammclib_bam_S32K14x/GDFLIB/F16/GDFLIB_FilterFIR_F16
      settings: RTWSystemCode=Inline
      mask Help: web([fileparts(which('ammclib_bam_S32K14x.slx')) '/../doc/S32K14XMCLUG.pdf'], '-browser')
      mask Display: pos = get_param(gcb, 'Position');width = pos(3) - pos(1); height = pos(4) - pos(2);tX=width/2;tY=height - 8;color('black');text(tX,tY, 'MLIB_VAdd_F16', 'horizontalAlignment', 'center');
  MLIB_VMac_F16 : Subsystem  TreatAsAtomicUnit=on  mask(MLIB_VMac_F16){}
      mask help: Dot product of 2-element vectors with saturated multiplication and modulo accumulation in 16-bit fixed-point fractional implementation. Refer to the AMMCLIB User's Guide for further details.
      mask init: same as ammclib_bam_S32K14x/GDFLIB/F16/GDFLIB_FilterFIR_F16
      settings: RTWSystemCode=Inline
      mask Help: web([fileparts(which('ammclib_bam_S32K14x.slx')) '/../doc/S32K14XMCLUG.pdf'], '-browser')
      mask Display: pos = get_param(gcb, 'Position');width = pos(3) - pos(1); height = pos(4) - pos(2);tX=width/2;tY=height - 8;color('black');text(tX,tY, 'MLIB_VMac_F16', 'horizontalAlignment', 'center');
  MLIB_VScale_F16 : Subsystem  TreatAsAtomicUnit=on  mask(MLIB_VScale_F16){}
      mask help: Multiplication of a vector and scalar in 16-bit fixed-point fractional implementation.
      mask init: same as ammclib_bam_S32K14x/GDFLIB/F16/GDFLIB_FilterFIR_F16
      settings: RTWSystemCode=Inline
      mask Help: web([fileparts(which('ammclib_bam_S32K14x.slx')) '/../doc/S32K14XMCLUG.pdf'], '-browser')
      mask Display: pos = get_param(gcb, 'Position');width = pos(3) - pos(1); height = pos(4) - pos(2);tX=width/2;tY=height - 8;color('black');text(tX,tY, 'MLIB_VScale_F16', 'horizontalAlignment', 'center');
  MLIB_VSub_F16 : Subsystem  TreatAsAtomicUnit=on  mask(MLIB_VSub_F16){}
      mask help: Vector substraction in 16-bit fixed-point fractional implementation.
      mask init: same as ammclib_bam_S32K14x/GDFLIB/F16/GDFLIB_FilterFIR_F16
      settings: RTWSystemCode=Inline
      mask Help: web([fileparts(which('ammclib_bam_S32K14x.slx')) '/../doc/S32K14XMCLUG.pdf'], '-browser')
      mask Display: pos = get_param(gcb, 'Position');width = pos(3) - pos(1); height = pos(4) - pos(2);tX=width/2;tY=height - 8;color('black');text(tX,tY, 'MLIB_VSub_F16', 'horizontalAlignment', 'center');
